simulink model "F550_Attitude_ctrl_SMC"  (R2024a)
settings: Solver=ode4  StartTime=0.0  StopTime=30  FixedStep=0.001  RelTol=1e-3
values from neighbouring files (symbols this model uses):
  r2d = 180/pi    (= 57.2957795131)    [Run_F550_Attitude_Sim.m]    (also in Run_F550_Attitude_Sim_SMC.m)
undefined symbols (not defined in the file or in its folder): Jxx, Jyy, Jzz, SampleTime
libraries: slpidlib x14, simulink x4, simulink_extras x3, matrix_library x1
(part 1 of 2)
settings Model: Creator=ADMIN  LastModifiedBy=UASG
settings DataIOCC: ExternalInput=getinputstruct(op_trim1)  InitialState=getstatestruct(op_trim1)
settings DebuggingCC: UnconnectedInputMsg=warning  UnconnectedOutputMsg=warning  UnconnectedLineMsg=warning  UnderSpecifiedDimensionMsg=warning
settings ModelReferenceCC: EnableRefExpFcnMdlSchedulingChecks=on
settings RTWCC: GPUComputeCapability=3.5  DLArmComputeVersion=19.05

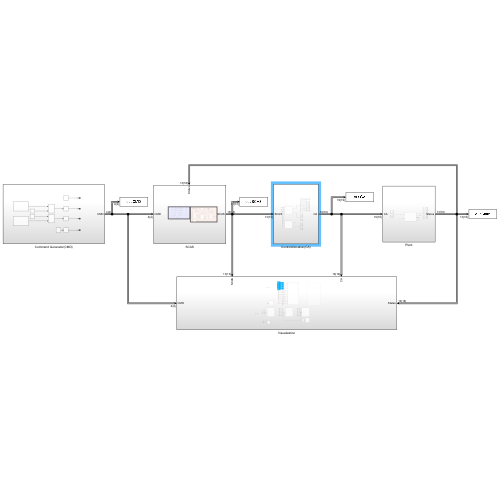
[thumbnail: Simulink's stored preview of the top-level diagram]
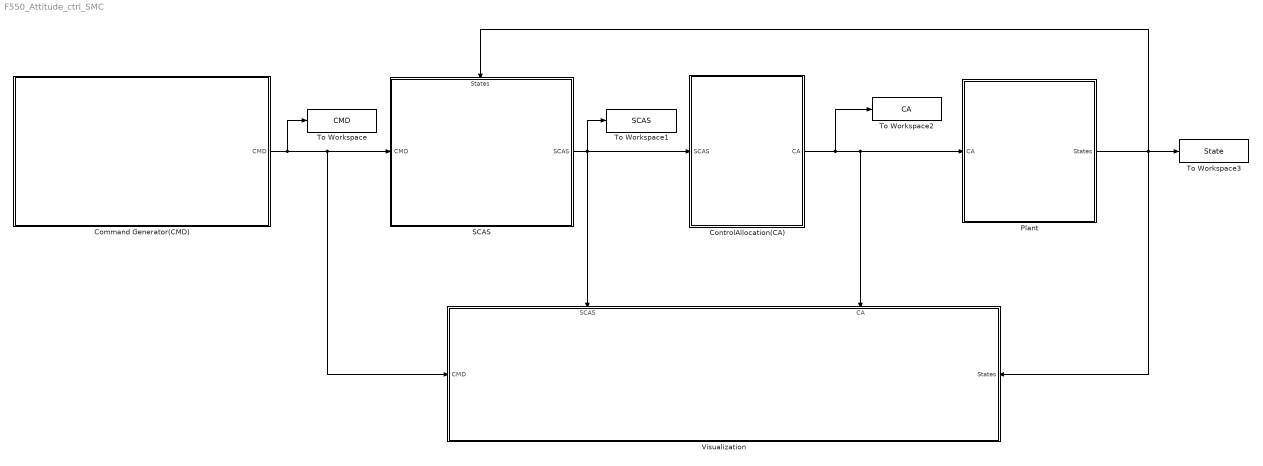
== system F550_Attitude_ctrl_SMC ==
  Command Generator(CMD) : Subsystem
  ControlAllocation(CA) : Subsystem
  Plant : Subsystem
  SCAS : Subsystem
      settings: PortSchema="{\"entries\":[{\"content\":{\"sides\":[{\"content\":{\"connectorIds\":[\"In1\"]},\"type\":\"ConnectorPlacement.EquallySpacedRectSide\",\"uuid\":\"45c0ffbb-c8f4-4882-ae07-b7c3e206befd\"},{\"content\":{\"connectorIds\":[\"Out1\"],\"side\":\"RIGHT\"},\"type\":\"ConnectorPlacement.EquallySpacedRectSide\",\"uuid\":\"fea4074d-042e-40e0-9516-e60d5ceca645\"},{\"content\":{\"connectorIds\":[\"In2\"],\"side\":\"TOP\"},\"type\":\"ConnectorPlacement.EquallySpacedRectSide\",\"uuid\":\"f0d79ab8-0f8c-4372-8ce2-381c487e77f0\"}]},\"type\":\"ConnectorPlacement.EquallySpacedConnector\",\"uuid\":\"9d757277-2882-485b-80f7-2c3f01a5660c\"}],\"packageUris\":[\"http://schema.mathworks.com/mf0/Connector/R2020b\"],\"version\":\"1.0\"}"
  To Workspace : ToWorkspace  VariableName=CMD  SaveFormat=Timeseries  SampleTime=-1
      settings: Save2DSignal=2-D array (concatenate along first dimension)
  To Workspace1 : ToWorkspace  VariableName=SCAS  SaveFormat=Timeseries  SampleTime=-1
      settings: Save2DSignal=2-D array (concatenate along first dimension)
  To Workspace2 : ToWorkspace  VariableName=CA  SaveFormat=Timeseries  SampleTime=-1
      settings: Save2DSignal=2-D array (concatenate along first dimension)
  To Workspace3 : ToWorkspace  VariableName=State  SaveFormat=Timeseries  SampleTime=-1
      settings: Save2DSignal=2-D array (concatenate along first dimension)
  Visualization : Subsystem
      settings: PortSchema="{\"entries\":[{\"content\":{\"sides\":[{\"content\":{\"connectorIds\":[\"In1\"]},\"type\":\"ConnectorPlacement.EquallySpacedRectSide\",\"uuid\":\"45c0ffbb-c8f4-4882-ae07-b7c3e206befd\"},{\"content\":{\"connectorIds\":[\"In4\"],\"side\":\"RIGHT\"},\"type\":\"ConnectorPlacement.EquallySpacedRectSide\",\"uuid\":\"fea4074d-042e-40e0-9516-e60d5ceca645\"},{\"content\":{\"connectorIds\":[\"In2\",\"In3\"],\"side\":\"TOP\"},\"type\":\"ConnectorPlacement.EquallySpacedRectSide\",\"uuid\":\"f0d79ab8-0f8c-4372-8ce2-381c487e77f0\"}]},\"type\":\"ConnectorPlacement.EquallySpacedConnector\",\"uuid\":\"9d757277-2882-485b-80f7-2c3f01a5660c\"}],\"packageUris\":[\"http://schema.mathworks.com/mf0/Connector/R2020b\"],\"version\":\"1.0\"}"
  wires:
  Command Generator(CMD)/1(CMD) -> To Workspace/1, Visualization/1(CMD), SCAS/1(CMD)
  Plant/1(States) -> SCAS/2(States), To Workspace3/1, Visualization/4(States)
  SCAS/1(SCAS) -> To Workspace1/1, ControlAllocation(CA)/1(SCAS), Visualization/2(SCAS)
  ControlAllocation(CA)/1(CA) -> To Workspace2/1, Visualization/3(CA), Plant/1(CA)

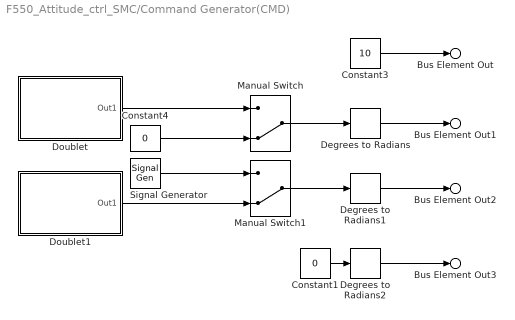
== system F550_Attitude_ctrl_SMC/Command Generator(CMD) ==
  Constant1 : Constant  Value=0
  Constant3 : Constant  Value=10
  Constant4 : Constant  Value=0
  Degrees to Radians : simulink_extras/Transformations/Degrees to Radians
  Degrees to Radians1 : simulink_extras/Transformations/Degrees to Radians
  Degrees to Radians2 : simulink_extras/Transformations/Degrees to Radians
  Doublet : Subsystem
  Doublet1 : Subsystem
  Manual Switch : ManualSwitch  CurrentSetting=0
  Manual Switch1 : ManualSwitch  CurrentSetting=0
  Signal Generator : SignalGenerator  Amplitude=10  Frequency=0.5
  Bus Element Out : Outport  PortName=CMD  Element=des_altitude
  Bus Element Out1 : Outport  PortName=CMD  Element=des_pitch
  Bus Element Out2 : Outport  PortName=CMD  Element=des_roll
  Bus Element Out3 : Outport  PortName=CMD  Element=des_yawrate
  wires:
  Constant1/1 -> Degrees to Radians2/1
  Degrees to Radians2/1 -> Bus Element Out3/1
  Constant3/1 -> Bus Element Out/1
  Degrees to Radians1/1 -> Bus Element Out2/1
  Degrees to Radians/1 -> Bus Element Out1/1
  Manual Switch/1 -> Degrees to Radians/1
  Constant4/1 -> Manual Switch/2
  Manual Switch1/1 -> Degrees to Radians1/1
  Signal Generator/1 -> Manual Switch1/1
  Doublet1/1(Out1) -> Manual Switch1/2
  Doublet/1(Out1) -> Manual Switch/1

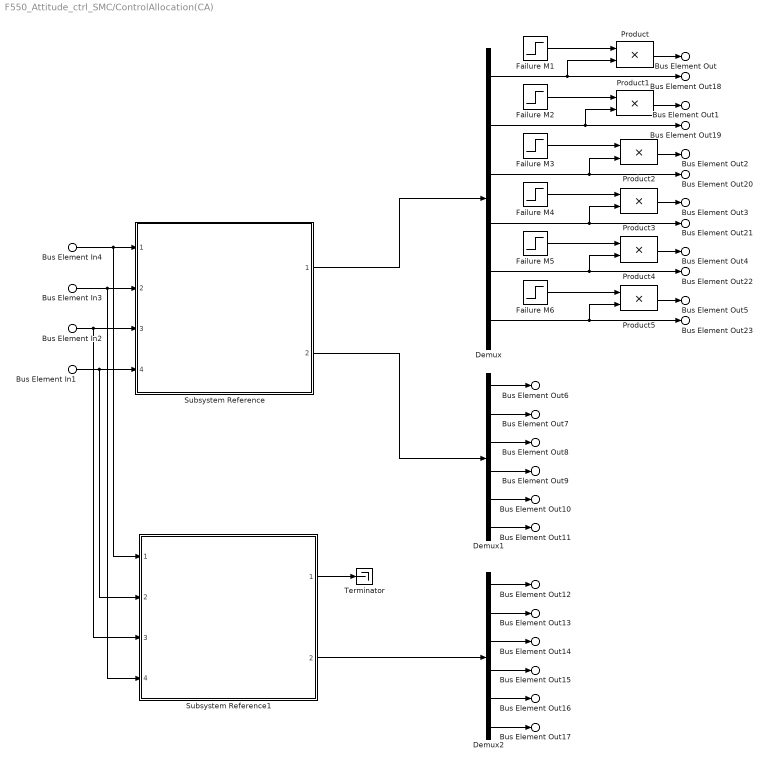
== system F550_Attitude_ctrl_SMC/ControlAllocation(CA) ==
  Bus Element In1 : Inport  PortName=SCAS  Element=tau_roll_smc
  Bus Element In2 : Inport  PortName=SCAS  Element=tau_pitch
  Bus Element In3 : Inport  PortName=SCAS  Element=tau_yaw
  Bus Element In4 : Inport  PortName=SCAS  Element=throttle
  " Failure M3" : Step  Time=23  Before=1  SampleTime=0
  " Failure M4" : Step  Time=23  Before=1  SampleTime=0
  " Failure M5" : Step  Time=23  Before=1  SampleTime=0
  " Failure M6 " : Step  Time=23  Before=1  SampleTime=0
  Demux : Demux  Outputs=6
  Demux1 : Demux  Outputs=6
  Demux2 : Demux  Outputs=6
  Failure M1 : Step  Time=23  Before=1  After=0.5  SampleTime=0
  Failure M2 : Step  Time=23  Before=1  SampleTime=0
  Product{,1..5} (6 alike) : Product
  Subsystem Reference : Subsystem  ReferencedSubsystem=F550_ControlAllocation_sub_ver2023b
  Subsystem Reference1 : Subsystem  ReferencedSubsystem=F550_Adam_CA
  Terminator : Terminator
  Bus Element Out : Outport  PortName=CA  Element=thr_m1
  Bus Element Out1 : Outport  PortName=CA  Element=thr_m2
  Bus Element Out2 : Outport  PortName=CA  Element=thr_m3
  Bus Element Out3 : Outport  PortName=CA  Element=thr_m4
  Bus Element Out4 : Outport  PortName=CA  Element=thr_m5
  Bus Element Out5 : Outport  PortName=CA  Element=thr_m6
  Bus Element Out6 : Outport  PortName=CA  Element=thr_before_saturation_m1
  Bus Element Out7 : Outport  PortName=CA  Element=thr_before_saturation_m2
  Bus Element Out8 : Outport  PortName=CA  Element=thr_before_saturation_m3
  Bus Element Out9 : Outport  PortName=CA  Element=thr_before_saturation_m4
  Bus Element Out10 : Outport  PortName=CA  Element=thr_before_saturation_m5
  Bus Element Out11 : Outport  PortName=CA  Element=thr_before_saturation_m6
  Bus Element Out12 : Outport  PortName=CA  Element=thr_adam_m1
  Bus Element Out13 : Outport  PortName=CA  Element=thr_adam_m2
  Bus Element Out14 : Outport  PortName=CA  Element=thr_adam_m3
  Bus Element Out15 : Outport  PortName=CA  Element=thr_adam_m4
  Bus Element Out16 : Outport  PortName=CA  Element=thr_adam_m5
  Bus Element Out17 : Outport  PortName=CA  Element=thr_adam_m6
  Bus Element Out18 : Outport  PortName=CA  Element=thr_m1_before_fail
  Bus Element Out19 : Outport  PortName=CA  Element=thr_m2_before_fail
  Bus Element Out20 : Outport  PortName=CA  Element=thr_m3_before_fail
  Bus Element Out21 : Outport  PortName=CA  Element=thr_m4_before_fail4
  Bus Element Out22 : Outport  PortName=CA  Element=thr_m5_before_fail
  Bus Element Out23 : Outport  PortName=CA  Element=thr_m6_before_fail
  wires:
  Bus Element In4/1 -> Subsystem Reference1/1, Subsystem Reference/1
  Bus Element In3/1 -> Subsystem Reference1/4, Subsystem Reference/2
  Bus Element In2/1 -> Subsystem Reference1/3, Subsystem Reference/3
  Bus Element In1/1 -> Subsystem Reference1/2, Subsystem Reference/4
  Subsystem Reference/2 -> Demux1/1
  Demux1/1 -> Bus Element Out6/1
  Demux1/2 -> Bus Element Out7/1
  Demux1/3 -> Bus Element Out8/1
  Demux1/4 -> Bus Element Out9/1
  Demux1/5 -> Bus Element Out10/1
  Demux1/6 -> Bus Element Out11/1
  Subsystem Reference1/2 -> Demux2/1
  Subsystem Reference1/1 -> Terminator/1
  Demux2/1 -> Bus Element Out12/1
  Demux2/2 -> Bus Element Out13/1
  Demux2/3 -> Bus Element Out14/1
  Demux2/4 -> Bus Element Out15/1
  Demux2/5 -> Bus Element Out16/1
  Demux2/6 -> Bus Element Out17/1
  Product/1 -> Bus Element Out/1
  Demux/1 -> Bus Element Out18/1, Product/2
  Failure M1/1 -> Product/1
  Subsystem Reference/1 -> Demux/1
  Demux/2 -> Product1/2, Bus Element Out19/1
  Product1/1 -> Bus Element Out1/1
  Failure M2/1 -> Product1/1
  Demux/3 -> Product2/2, Bus Element Out20/1
  Product2/1 -> Bus Element Out2/1
  " Failure M3"/1 -> Product2/1
  Demux/4 -> Bus Element Out21/1, Product3/2
  Product3/1 -> Bus Element Out3/1
  " Failure M4"/1 -> Product3/1
  Demux/5 -> Bus Element Out22/1, Product4/2
  Product4/1 -> Bus Element Out4/1
  " Failure M5"/1 -> Product4/1
  Demux/6 -> Bus Element Out23/1, Product5/2
  Product5/1 -> Bus Element Out5/1
  " Failure M6 "/1 -> Product5/1

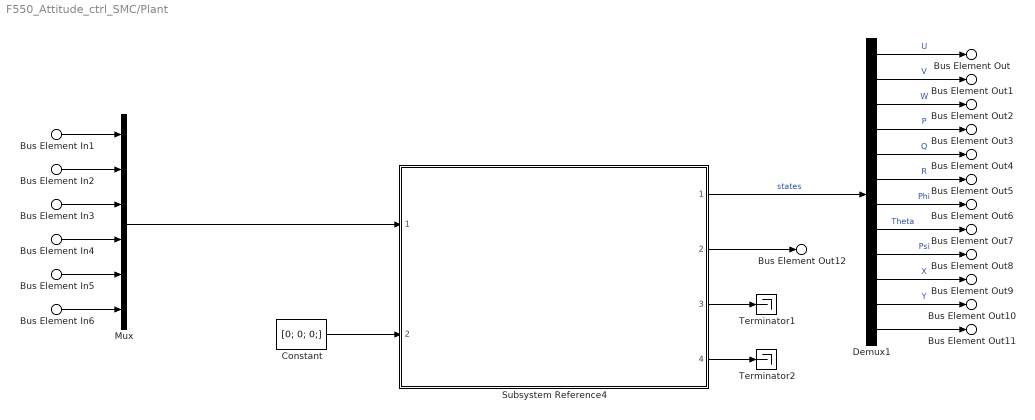
== system F550_Attitude_ctrl_SMC/Plant ==
  Bus Element In1 : Inport  PortName=CA  Element=thr_m1
  Bus Element In2 : Inport  PortName=CA  Element=thr_m2
  Bus Element In3 : Inport  PortName=CA  Element=thr_m3
  Bus Element In4 : Inport  PortName=CA  Element=thr_m4
  Bus Element In5 : Inport  PortName=CA  Element=thr_m5
  Bus Element In6 : Inport  PortName=CA  Element=thr_m6
  Constant : Constant  Value=[0; 0; 0;]
  Demux1 : Demux  Outputs=12
  Mux : Mux  Inputs=6
  Subsystem Reference4 : Subsystem  ReferencedSubsystem=F550_Dynamics_sub_ver2023b
  Terminator1 : Terminator
  Terminator2 : Terminator
  Bus Element Out : Outport  PortName=States  Element=u
  Bus Element Out1 : Outport  PortName=States  Element=v
  Bus Element Out2 : Outport  PortName=States  Element=w
  Bus Element Out3 : Outport  PortName=States  Element=p
  Bus Element Out4 : Outport  PortName=States  Element=q
  Bus Element Out5 : Outport  PortName=States  Element=r
  Bus Element Out6 : Outport  PortName=States  Element=phi
  Bus Element Out7 : Outport  PortName=States  Element=theta
  Bus Element Out8 : Outport  PortName=States  Element=psi
  Bus Element Out9 : Outport  PortName=States  Element=x
  Bus Element Out10 : Outport  PortName=States  Element=y
  Bus Element Out11 : Outport  PortName=States  Element=z
  Bus Element Out12 : Outport  PortName=States  Element=rpm
  wires:
  Subsystem Reference4/1 -> Demux1/1  "states"
  Demux1/1 -> Bus Element Out/1  "U"
  Demux1/2 -> Bus Element Out1/1  "V"
  Demux1/3 -> Bus Element Out2/1  "W"
  Demux1/4 -> Bus Element Out3/1  "P"
  Demux1/5 -> Bus Element Out4/1  "Q"
  Demux1/6 -> Bus Element Out5/1  "R"
  Demux1/7 -> Bus Element Out6/1  "Phi"
  Demux1/8 -> Bus Element Out7/1  "Theta"
  Demux1/9 -> Bus Element Out8/1  "Psi"
  Demux1/10 -> Bus Element Out9/1  "X"
  Demux1/11 -> Bus Element Out10/1  "Y"
  Demux1/12 -> Bus Element Out11/1
  Subsystem Reference4/2 -> Bus Element Out12/1
  Subsystem Reference4/3 -> Terminator1/1
  Subsystem Reference4/4 -> Terminator2/1
  Bus Element In1/1 -> Mux/1
  Bus Element In2/1 -> Mux/2
  Bus Element In3/1 -> Mux/3
  Bus Element In4/1 -> Mux/4
  Bus Element In5/1 -> Mux/5
  Bus Element In6/1 -> Mux/6
  Mux/1 -> Subsystem Reference4/1
  Constant/1 -> Subsystem Reference4/2

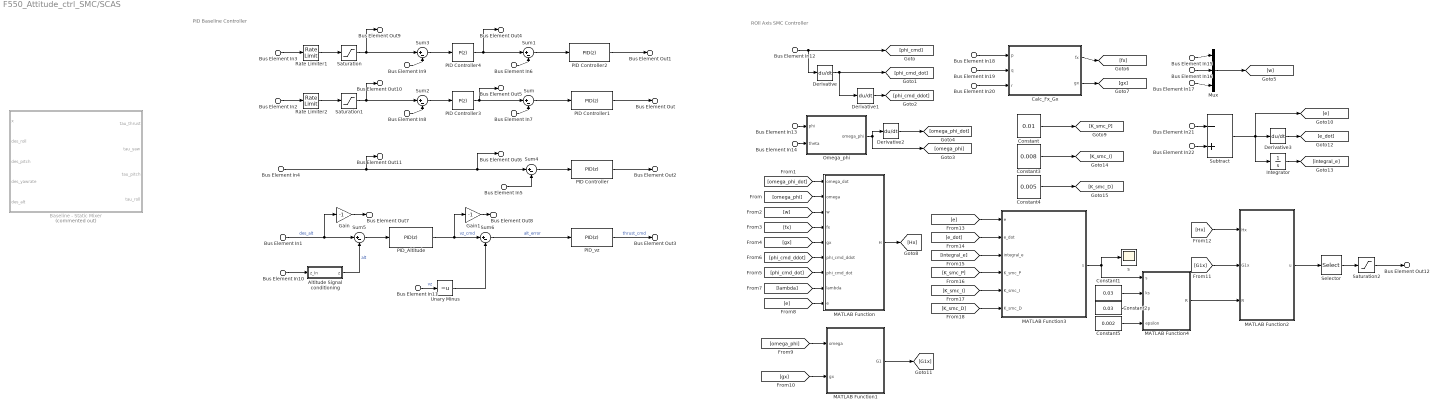
== system F550_Attitude_ctrl_SMC/SCAS ==
  note: ROll Axis SMC Controller
  note: PID Baseline Controller
  Bus Element In1 : Inport  PortName=CMD  Element=des_altitude
  Bus Element In2 : Inport  PortName=CMD  Element=des_pitch
  Bus Element In3 : Inport  PortName=CMD  Element=des_roll
  Bus Element In12 : Inport  PortName=CMD  Element=des_roll
  Bus Element In21 : Inport  PortName=CMD  Element=des_roll
  Bus Element In4 : Inport  PortName=CMD  Element=des_yawrate
  Bus Element In5 : Inport  Port=2  PortName=States  Element=r
  Bus Element In17 : Inport  Port=2  PortName=States  Element=r
  Bus Element In20 : Inport  Port=2  PortName=States  Element=r
  Bus Element In6 : Inport  Port=2  PortName=States  Element=p
  Bus Element In15 : Inport  Port=2  PortName=States  Element=p
  Bus Element In18 : Inport  Port=2  PortName=States  Element=p
  Bus Element In7 : Inport  Port=2  PortName=States  Element=q
  Bus Element In16 : Inport  Port=2  PortName=States  Element=q
  Bus Element In19 : Inport  Port=2  PortName=States  Element=q
  Bus Element In8 : Inport  Port=2  PortName=States  Element=theta
  Bus Element In14 : Inport  Port=2  PortName=States  Element=theta
  Bus Element In9 : Inport  Port=2  PortName=States  Element=phi
  Bus Element In13 : Inport  Port=2  PortName=States  Element=phi
  Bus Element In22 : Inport  Port=2  PortName=States  Element=phi
  Bus Element In10 : Inport  Port=2  PortName=States  Element=z
  Bus Element In11 : Inport  Port=2  PortName=States  Element=w
  Altitude Signal conditioning : Subsystem
  Baseline - Static Mixer : Subsystem  Commented=on
  Calc_Fx_Gx : Subsystem
  Constant : Constant  Value=0.01
  Constant1 : Constant  Value=0.03
  Constant2 : Constant  Value=0.03
  Constant3 : Constant  Value=0.008
  Constant4 : Constant  Value=0.005
  Constant5 : Constant  Value=0.002
  Derivative{,1..3} (4 alike) : Derivative
  Gain : Gain  Gain=-1
  Gain1 : Gain  Gain=-1
  Integrator : Integrator
  MATLAB Function : MATLAB Function  TreatAsAtomicUnit=on
  MATLAB Function1 : MATLAB Function  TreatAsAtomicUnit=on
  MATLAB Function2 : MATLAB Function  TreatAsAtomicUnit=on
  MATLAB Function3 : MATLAB Function  TreatAsAtomicUnit=on
  MATLAB Function4 : MATLAB Function  TreatAsAtomicUnit=on
  Mux : Mux  Inputs=3
  Omega_phi : MATLAB Function  TreatAsAtomicUnit=on
  PID Controller : slpidlib/PID Controller  Controller=PID  Form=Parallel  TimeDomain=Discrete-time  UseExternalTs=off  SampleTime=-1  IntegratorMethod=Forward Euler  FilterMethod=Forward Euler  ControllerParametersSource=internal  P=0.2  I=0.1  UseKiTs=off  D=0  UseExternalDerivativeSource=off  N=100  UseFilter=on  TunerSelectOption=Transfer Function Based (PID Tuner App)  InitialConditionSource=internal  InitialConditionForIntegrator=0  InitialConditionForFilter=0  DifferentiatorICPrevScaledInput=0  ExternalReset=none  TrackingMode=off  Kt=1  LimitOutput=off  SatLimitsSource=internal  UpperSaturationLimit=0.1  LowerSaturationLimit=-0.1  LinearizeAsGain=on  AntiWindupMode=clamping  Kb=1  LimitIntegrator=off  UpperIntegratorSaturationLimit=inf  LowerIntegratorSaturationLimit=-inf  POutMin=[]  POutMax=[]  IOutMin=[]  IOutMax=[]  DOutMin=[]  DOutMax=[]  NOutMin=[]  NOutMax=[]  SumOutMin=[]  SumOutMax=[]  SaturationOutMin=[]  SaturationOutMax=[]  PParamMin=[]  PParamMax=[]  IParamMin=[]  IParamMax=[]  DParamMin=[]  DParamMax=[]  NParamMin=[]  NParamMax=[]  KbParamMin=[]  KbParamMax=[]  KtParamMin=[]  KtParamMax=[]  KbOutMin=[]  KbOutMax=[]  KtOutMin=[]  KtOutMax=[]  IntegratorOutMin=[]  IntegratorOutMax=[]  FilterOutMin=[]  FilterOutMax=[]  SumI1OutMin=[]  SumI1OutMax=[]  SumI2OutMin=[]  SumI2OutMax=[]  SumI3OutMin=[]  SumI3OutMax=[]  SumI4OutMin=[]  SumI4OutMax=[]  SumDOutMin=[]  SumDOutMax=[]  DifferentiatorOutMin=[]  DifferentiatorOutMax=[]  FilterDiffOutCoefMin=[]  FilterDiffOutCoefMax=[]  ReciprocalOutMin=[]  ReciprocalOutMax=[]  SumDenOutMin=[]  SumDenOutMax=[]  SumNumOutMin=[]  SumNumOutMax=[]  DivideOutMin=[]  DivideOutMax=[]  UdiffTsProdOutMin=[]  UdiffTsProdOutMax=[]  NTsProdOutMin=[]  NTsProdOutMax=[]  UintegralTsProdOutMin=[]  UintegralTsProdOutMax=[]  UngainTsProdOutMin=[]  UngainTsProdOutMax=[]  ClampingZeroOutDataTypeStr=Inherit: Inherit via back propagation  ClampingZeroOutMin=[]  ClampingZeroOutMax=[]  FilterDenConstantOutDataTypeStr=Inherit: Inherit via back propagation  FilterDenConstantOutMin=[]  FilterDenConstantOutMax=[]  PCopyOutDataTypeStr=Inherit: Inherit via back propagation  PCopyOutMin=[]  PCopyOutMax=[]  NCopyOutDataTypeStr=Inherit: Inherit via back propagation  NCopyOutMin=[]  NCopyOutMax=[]  IntegratorContinuousStateAttributes=''  IntegratorStateMustResolveToSignalObject=off  IntegratorRTWStateStorageClass=Auto  FilterContinuousStateAttributes=''  FilterStateMustResolveToSignalObject=off  FilterRTWStateStorageClass=Auto  ParallelPVariant=InternalParameters  IdealPVariant=Disabled  IVariant=InternalParameters  DVariant=InternalParameters  IntegratorVariant=Discrete  SatVariant=Disabled  AWVariant=Passthrough  PCopyVariant=Disabled  TRVariant=Disabled  FdbkBlocksVariant=Forward  IdealPFdbkVariant=Disabled  SatFdbkVariant=Disabled  DerivativeFilterVariant=ForwardEulerFilter  NVariant=InternalParameters  NCopyVariant=Disabled  FilterICVariant=InternalICsFilter  IntegratorICVariant=InternalICs  ExternalResetVariant=Disabled  TRSumVariant=Passthrough  SumFdbkVariant=Disabled  SumVariant=Sum_PID  TsampFilterVariant=InternalTs  TsampNgainVariant=Passthrough  TsampIntegralVariant=Disabled_SignalSpec  ExternalSaturationOutDataTypeStr=Inherit: Same as second input  DerivativeSourceVariant=ErrorSignal
  PID Controller1 : slpidlib/PID Controller  Controller=PID  Form=Parallel  TimeDomain=Discrete-time  UseExternalTs=off  SampleTime=-1  IntegratorMethod=Forward Euler  FilterMethod=Forward Euler  ControllerParametersSource=internal  P=0.17  I=0.2  UseKiTs=off  D=0.006  UseExternalDerivativeSource=off  N=50  UseFilter=on  TunerSelectOption=Transfer Function Based (PID Tuner App)  InitialConditionSource=internal  InitialConditionForIntegrator=0  InitialConditionForFilter=0  DifferentiatorICPrevScaledInput=0  ExternalReset=none  TrackingMode=off  Kt=1  LimitOutput=off  SatLimitsSource=internal  UpperSaturationLimit=0.2  LowerSaturationLimit=-0.2  LinearizeAsGain=on  AntiWindupMode=clamping  Kb=1  LimitIntegrator=off  UpperIntegratorSaturationLimit=inf  LowerIntegratorSaturationLimit=-inf  POutMin=[]  POutMax=[]  IOutMin=[]  IOutMax=[]  DOutMin=[]  DOutMax=[]  NOutMin=[]  NOutMax=[]  SumOutMin=[]  SumOutMax=[]  SaturationOutMin=[]  SaturationOutMax=[]  PParamMin=[]  PParamMax=[]  IParamMin=[]  IParamMax=[]  DParamMin=[]  DParamMax=[]  NParamMin=[]  NParamMax=[]  KbParamMin=[]  KbParamMax=[]  KtParamMin=[]  KtParamMax=[]  KbOutMin=[]  KbOutMax=[]  KtOutMin=[]  KtOutMax=[]  IntegratorOutMin=[]  IntegratorOutMax=[]  FilterOutMin=[]  FilterOutMax=[]  SumI1OutMin=[]  SumI1OutMax=[]  SumI2OutMin=[]  SumI2OutMax=[]  SumI3OutMin=[]  SumI3OutMax=[]  SumI4OutMin=[]  SumI4OutMax=[]  SumDOutMin=[]  SumDOutMax=[]  DifferentiatorOutMin=[]  DifferentiatorOutMax=[]  FilterDiffOutCoefMin=[]  FilterDiffOutCoefMax=[]  ReciprocalOutMin=[]  ReciprocalOutMax=[]  SumDenOutMin=[]  SumDenOutMax=[]  SumNumOutMin=[]  SumNumOutMax=[]  DivideOutMin=[]  DivideOutMax=[]  UdiffTsProdOutMin=[]  UdiffTsProdOutMax=[]  NTsProdOutMin=[]  NTsProdOutMax=[]  UintegralTsProdOutMin=[]  UintegralTsProdOutMax=[]  UngainTsProdOutMin=[]  UngainTsProdOutMax=[]  ClampingZeroOutDataTypeStr=Inherit: Inherit via back propagation  ClampingZeroOutMin=[]  ClampingZeroOutMax=[]  FilterDenConstantOutDataTypeStr=Inherit: Inherit via back propagation  FilterDenConstantOutMin=[]  FilterDenConstantOutMax=[]  PCopyOutDataTypeStr=Inherit: Inherit via back propagation  PCopyOutMin=[]  PCopyOutMax=[]  NCopyOutDataTypeStr=Inherit: Inherit via back propagation  NCopyOutMin=[]  NCopyOutMax=[]  IntegratorContinuousStateAttributes=''  IntegratorStateMustResolveToSignalObject=off  IntegratorRTWStateStorageClass=Auto  FilterContinuousStateAttributes=''  FilterStateMustResolveToSignalObject=off  FilterRTWStateStorageClass=Auto  ParallelPVariant=InternalParameters  IdealPVariant=Disabled  IVariant=InternalParameters  DVariant=InternalParameters  IntegratorVariant=Discrete  SatVariant=Disabled  AWVariant=Passthrough  PCopyVariant=Disabled  TRVariant=Disabled  FdbkBlocksVariant=Forward  IdealPFdbkVariant=Disabled  SatFdbkVariant=Disabled  DerivativeFilterVariant=ForwardEulerFilter  NVariant=InternalParameters  NCopyVariant=Disabled  FilterICVariant=InternalICsFilter  IntegratorICVariant=InternalICs  ExternalResetVariant=Disabled  TRSumVariant=Passthrough  SumFdbkVariant=Disabled  SumVariant=Sum_PID  TsampFilterVariant=InternalTs  TsampNgainVariant=Passthrough  TsampIntegralVariant=Disabled_SignalSpec  ExternalSaturationOutDataTypeStr=Inherit: Same as second input  DerivativeSourceVariant=ErrorSignal
  PID Controller2 : slpidlib/PID Controller  Controller=PID  Form=Parallel  TimeDomain=Discrete-time  UseExternalTs=off  SampleTime=-1  IntegratorMethod=Forward Euler  FilterMethod=Forward Euler  ControllerParametersSource=internal  P=0.17  I=0.2  UseKiTs=off  D=0.006  UseExternalDerivativeSource=off  N=50  UseFilter=on  TunerSelectOption=Transfer Function Based (PID Tuner App)  InitialConditionSource=internal  InitialConditionForIntegrator=0  InitialConditionForFilter=0  DifferentiatorICPrevScaledInput=0  ExternalReset=none  TrackingMode=off  Kt=1  LimitOutput=off  SatLimitsSource=internal  UpperSaturationLimit=0.2  LowerSaturationLimit=-0.2  LinearizeAsGain=on  AntiWindupMode=clamping  Kb=1  LimitIntegrator=off  UpperIntegratorSaturationLimit=inf  LowerIntegratorSaturationLimit=-inf  POutMin=[]  POutMax=[]  IOutMin=[]  IOutMax=[]  DOutMin=[]  DOutMax=[]  NOutMin=[]  NOutMax=[]  SumOutMin=[]  SumOutMax=[]  SaturationOutMin=[]  SaturationOutMax=[]  PParamMin=[]  PParamMax=[]  IParamMin=[]  IParamMax=[]  DParamMin=[]  DParamMax=[]  NParamMin=[]  NParamMax=[]  KbParamMin=[]  KbParamMax=[]  KtParamMin=[]  KtParamMax=[]  KbOutMin=[]  KbOutMax=[]  KtOutMin=[]  KtOutMax=[]  IntegratorOutMin=[]  IntegratorOutMax=[]  FilterOutMin=[]  FilterOutMax=[]  SumI1OutMin=[]  SumI1OutMax=[]  SumI2OutMin=[]  SumI2OutMax=[]  SumI3OutMin=[]  SumI3OutMax=[]  SumI4OutMin=[]  SumI4OutMax=[]  SumDOutMin=[]  SumDOutMax=[]  DifferentiatorOutMin=[]  DifferentiatorOutMax=[]  FilterDiffOutCoefMin=[]  FilterDiffOutCoefMax=[]  ReciprocalOutMin=[]  ReciprocalOutMax=[]  SumDenOutMin=[]  SumDenOutMax=[]  SumNumOutMin=[]  SumNumOutMax=[]  DivideOutMin=[]  DivideOutMax=[]  UdiffTsProdOutMin=[]  UdiffTsProdOutMax=[]  NTsProdOutMin=[]  NTsProdOutMax=[]  UintegralTsProdOutMin=[]  UintegralTsProdOutMax=[]  UngainTsProdOutMin=[]  UngainTsProdOutMax=[]  ClampingZeroOutDataTypeStr=Inherit: Inherit via back propagation  ClampingZeroOutMin=[]  ClampingZeroOutMax=[]  FilterDenConstantOutDataTypeStr=Inherit: Inherit via back propagation  FilterDenConstantOutMin=[]  FilterDenConstantOutMax=[]  PCopyOutDataTypeStr=Inherit: Inherit via back propagation  PCopyOutMin=[]  PCopyOutMax=[]  NCopyOutDataTypeStr=Inherit: Inherit via back propagation  NCopyOutMin=[]  NCopyOutMax=[]  IntegratorContinuousStateAttributes=''  IntegratorStateMustResolveToSignalObject=off  IntegratorRTWStateStorageClass=Auto  FilterContinuousStateAttributes=''  FilterStateMustResolveToSignalObject=off  FilterRTWStateStorageClass=Auto  ParallelPVariant=InternalParameters  IdealPVariant=Disabled  IVariant=InternalParameters  DVariant=InternalParameters  IntegratorVariant=Discrete  SatVariant=Disabled  AWVariant=Passthrough  PCopyVariant=Disabled  TRVariant=Disabled  FdbkBlocksVariant=Forward  IdealPFdbkVariant=Disabled  SatFdbkVariant=Disabled  DerivativeFilterVariant=ForwardEulerFilter  NVariant=InternalParameters  NCopyVariant=Disabled  FilterICVariant=InternalICsFilter  IntegratorICVariant=InternalICs  ExternalResetVariant=Disabled  TRSumVariant=Passthrough  SumFdbkVariant=Disabled  SumVariant=Sum_PID  TsampFilterVariant=InternalTs  TsampNgainVariant=Passthrough  TsampIntegralVariant=Disabled_SignalSpec  ExternalSaturationOutDataTypeStr=Inherit: Same as second input  DerivativeSourceVariant=ErrorSignal
  PID Controller3 : slpidlib/PID Controller  Controller=P  Form=Parallel  TimeDomain=Discrete-time  UseExternalTs=off  SampleTime=-1  IntegratorMethod=Forward Euler  FilterMethod=Forward Euler  ControllerParametersSource=internal  P=7.0  I=1  UseKiTs=off  D=0  UseExternalDerivativeSource=off  N=100  UseFilter=on  TunerSelectOption=Transfer Function Based (PID Tuner App)  InitialConditionSource=internal  InitialConditionForIntegrator=0  InitialConditionForFilter=0  DifferentiatorICPrevScaledInput=0  ExternalReset=none  TrackingMode=off  Kt=1  LimitOutput=off  SatLimitsSource=internal  UpperSaturationLimit=inf  LowerSaturationLimit=-inf  LinearizeAsGain=on  AntiWindupMode=none  Kb=1  LimitIntegrator=off  UpperIntegratorSaturationLimit=inf  LowerIntegratorSaturationLimit=-inf  POutMin=[]  POutMax=[]  IOutMin=[]  IOutMax=[]  DOutMin=[]  DOutMax=[]  NOutMin=[]  NOutMax=[]  SumOutMin=[]  SumOutMax=[]  SaturationOutMin=[]  SaturationOutMax=[]  PParamMin=[]  PParamMax=[]  IParamMin=[]  IParamMax=[]  DParamMin=[]  DParamMax=[]  NParamMin=[]  NParamMax=[]  KbParamMin=[]  KbParamMax=[]  KtParamMin=[]  KtParamMax=[]  KbOutMin=[]  KbOutMax=[]  KtOutMin=[]  KtOutMax=[]  IntegratorOutMin=[]  IntegratorOutMax=[]  FilterOutMin=[]  FilterOutMax=[]  SumI1OutMin=[]  SumI1OutMax=[]  SumI2OutMin=[]  SumI2OutMax=[]  SumI3OutMin=[]  SumI3OutMax=[]  SumI4OutMin=[]  SumI4OutMax=[]  SumDOutMin=[]  SumDOutMax=[]  DifferentiatorOutMin=[]  DifferentiatorOutMax=[]  FilterDiffOutCoefMin=[]  FilterDiffOutCoefMax=[]  ReciprocalOutMin=[]  ReciprocalOutMax=[]  SumDenOutMin=[]  SumDenOutMax=[]  SumNumOutMin=[]  SumNumOutMax=[]  DivideOutMin=[]  DivideOutMax=[]  UdiffTsProdOutMin=[]  UdiffTsProdOutMax=[]  NTsProdOutMin=[]  NTsProdOutMax=[]  UintegralTsProdOutMin=[]  UintegralTsProdOutMax=[]  UngainTsProdOutMin=[]  UngainTsProdOutMax=[]  ClampingZeroOutDataTypeStr=Inherit: Inherit via back propagation  ClampingZeroOutMin=[]  ClampingZeroOutMax=[]  FilterDenConstantOutDataTypeStr=Inherit: Inherit via back propagation  FilterDenConstantOutMin=[]  FilterDenConstantOutMax=[]  PCopyOutDataTypeStr=Inherit: Inherit via back propagation  PCopyOutMin=[]  PCopyOutMax=[]  NCopyOutDataTypeStr=Inherit: Inherit via back propagation  NCopyOutMin=[]  NCopyOutMax=[]  IntegratorContinuousStateAttributes=''  IntegratorStateMustResolveToSignalObject=off  IntegratorRTWStateStorageClass=Auto  FilterContinuousStateAttributes=''  FilterStateMustResolveToSignalObject=off  FilterRTWStateStorageClass=Auto  ParallelPVariant=InternalParameters  IdealPVariant=Disabled  IVariant=Disabled  DVariant=Disabled  IntegratorVariant=Disabled  SatVariant=Disabled  AWVariant=Disabled  PCopyVariant=Disabled  TRVariant=Disabled  FdbkBlocksVariant=Forward  IdealPFdbkVariant=Disabled  SatFdbkVariant=Disabled  DerivativeFilterVariant=Disabled  NVariant=Disabled  NCopyVariant=Disabled_SignalSpec  FilterICVariant=Disabled  IntegratorICVariant=Disabled  ExternalResetVariant=Disabled  TRSumVariant=Passthrough  SumFdbkVariant=Disabled  SumVariant=Passthrough_P  TsampFilterVariant=InternalTs  TsampNgainVariant=Passthrough  TsampIntegralVariant=Disabled_SignalSpec  ExternalSaturationOutDataTypeStr=Inherit: Same as second input  DerivativeSourceVariant=Disabled
  PID Controller4 : slpidlib/PID Controller  Controller=P  Form=Parallel  TimeDomain=Discrete-time  UseExternalTs=off  SampleTime=-1  IntegratorMethod=Forward Euler  FilterMethod=Forward Euler  ControllerParametersSource=internal  P=7.0  I=1  UseKiTs=off  D=0  UseExternalDerivativeSource=off  N=100  UseFilter=on  TunerSelectOption=Transfer Function Based (PID Tuner App)  InitialConditionSource=internal  InitialConditionForIntegrator=0  InitialConditionForFilter=0  DifferentiatorICPrevScaledInput=0  ExternalReset=none  TrackingMode=off  Kt=1  LimitOutput=off  SatLimitsSource=internal  UpperSaturationLimit=inf  LowerSaturationLimit=-inf  LinearizeAsGain=on  AntiWindupMode=none  Kb=1  LimitIntegrator=off  UpperIntegratorSaturationLimit=inf  LowerIntegratorSaturationLimit=-inf  POutMin=[]  POutMax=[]  IOutMin=[]  IOutMax=[]  DOutMin=[]  DOutMax=[]  NOutMin=[]  NOutMax=[]  SumOutMin=[]  SumOutMax=[]  SaturationOutMin=[]  SaturationOutMax=[]  PParamMin=[]  PParamMax=[]  IParamMin=[]  IParamMax=[]  DParamMin=[]  DParamMax=[]  NParamMin=[]  NParamMax=[]  KbParamMin=[]  KbParamMax=[]  KtParamMin=[]  KtParamMax=[]  KbOutMin=[]  KbOutMax=[]  KtOutMin=[]  KtOutMax=[]  IntegratorOutMin=[]  IntegratorOutMax=[]  FilterOutMin=[]  FilterOutMax=[]  SumI1OutMin=[]  SumI1OutMax=[]  SumI2OutMin=[]  SumI2OutMax=[]  SumI3OutMin=[]  SumI3OutMax=[]  SumI4OutMin=[]  SumI4OutMax=[]  SumDOutMin=[]  SumDOutMax=[]  DifferentiatorOutMin=[]  DifferentiatorOutMax=[]  FilterDiffOutCoefMin=[]  FilterDiffOutCoefMax=[]  ReciprocalOutMin=[]  ReciprocalOutMax=[]  SumDenOutMin=[]  SumDenOutMax=[]  SumNumOutMin=[]  SumNumOutMax=[]  DivideOutMin=[]  DivideOutMax=[]  UdiffTsProdOutMin=[]  UdiffTsProdOutMax=[]  NTsProdOutMin=[]  NTsProdOutMax=[]  UintegralTsProdOutMin=[]  UintegralTsProdOutMax=[]  UngainTsProdOutMin=[]  UngainTsProdOutMax=[]  ClampingZeroOutDataTypeStr=Inherit: Inherit via back propagation  ClampingZeroOutMin=[]  ClampingZeroOutMax=[]  FilterDenConstantOutDataTypeStr=Inherit: Inherit via back propagation  FilterDenConstantOutMin=[]  FilterDenConstantOutMax=[]  PCopyOutDataTypeStr=Inherit: Inherit via back propagation  PCopyOutMin=[]  PCopyOutMax=[]  NCopyOutDataTypeStr=Inherit: Inherit via back propagation  NCopyOutMin=[]  NCopyOutMax=[]  IntegratorContinuousStateAttributes=''  IntegratorStateMustResolveToSignalObject=off  IntegratorRTWStateStorageClass=Auto  FilterContinuousStateAttributes=''  FilterStateMustResolveToSignalObject=off  FilterRTWStateStorageClass=Auto  ParallelPVariant=InternalParameters  IdealPVariant=Disabled  IVariant=Disabled  DVariant=Disabled  IntegratorVariant=Disabled  SatVariant=Disabled  AWVariant=Disabled  PCopyVariant=Disabled  TRVariant=Disabled  FdbkBlocksVariant=Forward  IdealPFdbkVariant=Disabled  SatFdbkVariant=Disabled  DerivativeFilterVariant=Disabled  NVariant=Disabled  NCopyVariant=Disabled_SignalSpec  FilterICVariant=Disabled  IntegratorICVariant=Disabled  ExternalResetVariant=Disabled  TRSumVariant=Passthrough  SumFdbkVariant=Disabled  SumVariant=Passthrough_P  TsampFilterVariant=InternalTs  TsampNgainVariant=Passthrough  TsampIntegralVariant=Disabled_SignalSpec  ExternalSaturationOutDataTypeStr=Inherit: Same as second input  DerivativeSourceVariant=Disabled
  PID_Altitude : slpidlib/PID Controller  Controller=PID  Form=Parallel  TimeDomain=Discrete-time  UseExternalTs=off  SampleTime=-1  IntegratorMethod=Backward Euler  FilterMethod=Forward Euler  ControllerParametersSource=internal  P=1.5  I=0.01  UseKiTs=off  D=0.01  UseExternalDerivativeSource=off  N=10  UseFilter=on  TunerSelectOption=Transfer Function Based (PID Tuner App)  InitialConditionSource=internal  InitialConditionForIntegrator=0  InitialConditionForFilter=0  DifferentiatorICPrevScaledInput=0  ExternalReset=none  TrackingMode=off  Kt=1  LimitOutput=on  SatLimitsSource=internal  UpperSaturationLimit=2  LowerSaturationLimit=-2  LinearizeAsGain=off  AntiWindupMode=clamping  Kb=1  LimitIntegrator=off  UpperIntegratorSaturationLimit=inf  LowerIntegratorSaturationLimit=-inf  POutMin=[]  POutMax=[]  IOutMin=[]  IOutMax=[]  DOutMin=[]  DOutMax=[]  NOutMin=[]  NOutMax=[]  SumOutMin=[]  SumOutMax=[]  SaturationOutMin=[]  SaturationOutMax=[]  PParamMin=[]  PParamMax=[]  IParamMin=[]  IParamMax=[]  DParamMin=[]  DParamMax=[]  NParamMin=[]  NParamMax=[]  KbParamMin=[]  KbParamMax=[]  KtParamMin=[]  KtParamMax=[]  KbOutMin=[]  KbOutMax=[]  KtOutMin=[]  KtOutMax=[]  IntegratorOutMin=[]  IntegratorOutMax=[]  FilterOutMin=[]  FilterOutMax=[]  SumI1OutMin=[]  SumI1OutMax=[]  SumI2OutMin=[]  SumI2OutMax=[]  SumI3OutMin=[]  SumI3OutMax=[]  SumI4OutMin=[]  SumI4OutMax=[]  SumDOutMin=[]  SumDOutMax=[]  DifferentiatorOutMin=[]  DifferentiatorOutMax=[]  FilterDiffOutCoefMin=[]  FilterDiffOutCoefMax=[]  ReciprocalOutMin=[]  ReciprocalOutMax=[]  SumDenOutMin=[]  SumDenOutMax=[]  SumNumOutMin=[]  SumNumOutMax=[]  DivideOutMin=[]  DivideOutMax=[]  UdiffTsProdOutMin=[]  UdiffTsProdOutMax=[]  NTsProdOutMin=[]  NTsProdOutMax=[]  UintegralTsProdOutMin=[]  UintegralTsProdOutMax=[]  UngainTsProdOutMin=[]  UngainTsProdOutMax=[]  ClampingZeroOutDataTypeStr=Inherit: Inherit via back propagation  ClampingZeroOutMin=[]  ClampingZeroOutMax=[]  FilterDenConstantOutDataTypeStr=Inherit: Inherit via back propagation  FilterDenConstantOutMin=[]  FilterDenConstantOutMax=[]  PCopyOutDataTypeStr=Inherit: Inherit via back propagation  PCopyOutMin=[]  PCopyOutMax=[]  NCopyOutDataTypeStr=Inherit: Inherit via back propagation  NCopyOutMin=[]  NCopyOutMax=[]  IntegratorContinuousStateAttributes=''  IntegratorStateMustResolveToSignalObject=off  IntegratorRTWStateStorageClass=Auto  FilterContinuousStateAttributes=''  FilterStateMustResolveToSignalObject=off  FilterRTWStateStorageClass=Auto  ParallelPVariant=InternalParameters  IdealPVariant=Disabled  IVariant=InternalParameters  DVariant=InternalParameters  IntegratorVariant=Discrete  SatVariant=Enabled  AWVariant=DiscClampingParallel  PCopyVariant=Disabled  TRVariant=Disabled  FdbkBlocksVariant=Feedback  IdealPFdbkVariant=Passthrough  SatFdbkVariant=Passthrough  DerivativeFilterVariant=ForwardEulerFilter  NVariant=InternalParameters  NCopyVariant=Disabled  FilterICVariant=InternalICsFilter  IntegratorICVariant=InternalICs  ExternalResetVariant=Disabled  TRSumVariant=Passthrough  SumFdbkVariant=Enabled  SumVariant=Sum_PID  TsampFilterVariant=InternalTs  TsampNgainVariant=Passthrough  TsampIntegralVariant=Disabled_SignalSpec  ExternalSaturationOutDataTypeStr=Inherit: Same as second input  DerivativeSourceVariant=ErrorSignal
  PID_vz : slpidlib/PID Controller  Controller=PID  Form=Parallel  TimeDomain=Discrete-time  UseExternalTs=off  SampleTime=-1  IntegratorMethod=Backward Euler  FilterMethod=Forward Euler  ControllerParametersSource=internal  P=0.5  I=0.1  UseKiTs=off  D=0.05  UseExternalDerivativeSource=off  N=10  UseFilter=on  TunerSelectOption=Transfer Function Based (PID Tuner App)  InitialConditionSource=internal  InitialConditionForIntegrator=0  InitialConditionForFilter=0  DifferentiatorICPrevScaledInput=0  ExternalReset=none  TrackingMode=off  Kt=1  LimitOutput=on  SatLimitsSource=internal  UpperSaturationLimit=1  LowerSaturationLimit=0  LinearizeAsGain=off  AntiWindupMode=clamping  Kb=1  LimitIntegrator=off  UpperIntegratorSaturationLimit=inf  LowerIntegratorSaturationLimit=-inf  POutMin=[]  POutMax=[]  IOutMin=[]  IOutMax=[]  DOutMin=[]  DOutMax=[]  NOutMin=[]  NOutMax=[]  SumOutMin=[]  SumOutMax=[]  SaturationOutMin=[]  SaturationOutMax=[]  PParamMin=[]  PParamMax=[]  IParamMin=[]  IParamMax=[]  DParamMin=[]  DParamMax=[]  NParamMin=[]  NParamMax=[]  KbParamMin=[]  KbParamMax=[]  KtParamMin=[]  KtParamMax=[]  KbOutMin=[]  KbOutMax=[]  KtOutMin=[]  KtOutMax=[]  IntegratorOutMin=[]  IntegratorOutMax=[]  FilterOutMin=[]  FilterOutMax=[]  SumI1OutMin=[]  SumI1OutMax=[]  SumI2OutMin=[]  SumI2OutMax=[]  SumI3OutMin=[]  SumI3OutMax=[]  SumI4OutMin=[]  SumI4OutMax=[]  SumDOutMin=[]  SumDOutMax=[]  DifferentiatorOutMin=[]  DifferentiatorOutMax=[]  FilterDiffOutCoefMin=[]  FilterDiffOutCoefMax=[]  ReciprocalOutMin=[]  ReciprocalOutMax=[]  SumDenOutMin=[]  SumDenOutMax=[]  SumNumOutMin=[]  SumNumOutMax=[]  DivideOutMin=[]  DivideOutMax=[]  UdiffTsProdOutMin=[]  UdiffTsProdOutMax=[]  NTsProdOutMin=[]  NTsProdOutMax=[]  UintegralTsProdOutMin=[]  UintegralTsProdOutMax=[]  UngainTsProdOutMin=[]  UngainTsProdOutMax=[]  ClampingZeroOutDataTypeStr=Inherit: Inherit via back propagation  ClampingZeroOutMin=[]  ClampingZeroOutMax=[]  FilterDenConstantOutDataTypeStr=Inherit: Inherit via back propagation  FilterDenConstantOutMin=[]  FilterDenConstantOutMax=[]  PCopyOutDataTypeStr=Inherit: Inherit via back propagation  PCopyOutMin=[]  PCopyOutMax=[]  NCopyOutDataTypeStr=Inherit: Inherit via back propagation  NCopyOutMin=[]  NCopyOutMax=[]  IntegratorContinuousStateAttributes=''  IntegratorStateMustResolveToSignalObject=off  IntegratorRTWStateStorageClass=Auto  FilterContinuousStateAttributes=''  FilterStateMustResolveToSignalObject=off  FilterRTWStateStorageClass=Auto  ParallelPVariant=InternalParameters  IdealPVariant=Disabled  IVariant=InternalParameters  DVariant=InternalParameters  IntegratorVariant=Discrete  SatVariant=Enabled  AWVariant=DiscClampingParallel  PCopyVariant=Disabled  TRVariant=Disabled  FdbkBlocksVariant=Feedback  IdealPFdbkVariant=Passthrough  SatFdbkVariant=Passthrough  DerivativeFilterVariant=ForwardEulerFilter  NVariant=InternalParameters  NCopyVariant=Disabled  FilterICVariant=InternalICsFilter  IntegratorICVariant=InternalICs  ExternalResetVariant=Disabled  TRSumVariant=Passthrough  SumFdbkVariant=Enabled  SumVariant=Sum_PID  TsampFilterVariant=InternalTs  TsampNgainVariant=Passthrough  TsampIntegralVariant=Disabled_SignalSpec  ExternalSaturationOutDataTypeStr=Inherit: Same as second input  DerivativeSourceVariant=ErrorSignal
  Rate Limiter1 : RateLimiter  RisingSlewLimit=180*pi/180  FallingSlewLimit=-180*pi/180  SampleTimeMode=inherited
  Rate Limiter2 : RateLimiter  RisingSlewLimit=180*pi/180  FallingSlewLimit=-180*pi/180  SampleTimeMode=inherited
  Saturation : Saturate  UpperLimit=20*pi/180  LowerLimit=-20*pi/180
  Saturation1 : Saturate  UpperLimit=20*pi/180  LowerLimit=-20*pi/180
  Saturation2 : Saturate
  Selector : Selector  InputPortWidth=3  IndexOptions=Index vector (dialog)  Indices=1  OutputSizes=1
  Subtract : Sum  Inputs=-+
  Sum{,1..6} (7 alike) : Sum  Inputs=|+-
  Unary Minus : UnaryMinus
  s : Scope
  Bus Element Out : Outport  PortName=SCAS  Element=tau_pitch
  Bus Element Out1 : Outport  PortName=SCAS  Element=tau_roll
  Bus Element Out2 : Outport  PortName=SCAS  Element=tau_yaw
  Bus Element Out3 : Outport  PortName=SCAS  Element=throttle
  Bus Element Out4 : Outport  PortName=SCAS  Element=p_cmd
  Bus Element Out5 : Outport  PortName=SCAS  Element=q_cmd
  Bus Element Out6 : Outport  PortName=SCAS  Element=r_cmd
  Bus Element Out7 : Outport  PortName=SCAS  Element=z_cmd
  Bus Element Out8 : Outport  PortName=SCAS  Element=w_cmd
  Bus Element Out9 : Outport  PortName=SCAS  Element=phi_cmd
  Bus Element Out10 : Outport  PortName=SCAS  Element=theta_cmd
  Bus Element Out11 : Outport  PortName=SCAS  Element=psi_cmd
  Bus Element Out12 : Outport  PortName=SCAS  Element=tau_roll_smc
  wires:
  Bus Element In2/1 -> Rate Limiter2/1
  Bus Element In4/1 -> Bus Element Out11/1, Bus Element Out6/1, Sum4/1
  Bus Element In3/1 -> Rate Limiter1/1
  PID Controller4/1 -> Bus Element Out4/1, Sum1/1
  Sum3/1 -> PID Controller4/1
  PID Controller1/1 -> Bus Element Out/1
  Saturation1/1 -> Bus Element Out10/1, Sum2/1
  Sum2/1 -> PID Controller3/1
  PID Controller3/1 -> Bus Element Out5/1, Sum/1
  Saturation/1 -> Sum3/1, Bus Element Out9/1
  Rate Limiter2/1 -> Saturation1/1
  Sum/1 -> PID Controller1/1
  Sum1/1 -> PID Controller2/1
  Rate Limiter1/1 -> Saturation/1
  PID Controller/1 -> Bus Element Out2/1
  Sum4/1 -> PID Controller/1
  Gain/1 -> Bus Element Out7/1
  Bus Element In11/1 -> Unary Minus/1  "vz"
  Gain1/1 -> Bus Element Out8/1
  Unary Minus/1 -> Sum6/2
  Altitude Signal conditioning/1(z) -> Sum5/2  "alt"
  Sum6/1 -> PID_vz/1  "alt_error"
  Bus Element In1/1 -> Gain/1, Sum5/1  "des_alt"
  Bus Element In10/1 -> Altitude Signal conditioning/1(z_In)
  Sum5/1 -> PID_Altitude/1
  PID_Altitude/1 -> Gain1/1, Sum6/1  "vz_cmd"
  PID_vz/1 -> Bus Element Out3/1  "thrust_cmd"
  Bus Element In5/1 -> Sum4/2
  Bus Element In6/1 -> Sum1/2
  Bus Element In7/1 -> Sum/2
  Bus Element In8/1 -> Sum2/2
  Bus Element In9/1 -> Sum3/2
  Bus Element In12/1 -> [phi_cmd], Derivative/1
  Derivative/1 -> [phi_cmd_dot], Derivative1/1
  Derivative1/1 -> [phi_cmd_ddot]
  Bus Element In13/1 -> Omega_phi/1(phi)
  Bus Element In14/1 -> Omega_phi/2(theta)
  Omega_phi/1(omega_phi) -> Derivative2/1, [omega_phi]
  Derivative2/1 -> [omega_phi_dot]
  Bus Element In15/1 -> Mux/1
  Bus Element In16/1 -> Mux/2
  Bus Element In17/1 -> Mux/3
  Mux/1 -> [w]
  Bus Element In18/1 -> Calc_Fx_Gx/1(p)
  Bus Element In19/1 -> Calc_Fx_Gx/2(q)
  Bus Element In20/1 -> Calc_Fx_Gx/3(r)
  Calc_Fx_Gx/1(fx) -> [fx]
  Calc_Fx_Gx/2(gx) -> [gx]
  MATLAB Function/1(H) -> [Hx]
  [omega_phi_dot] -> MATLAB Function/1(omega_dot)
  [omega_phi] -> MATLAB Function/2(omega)
  [w] -> MATLAB Function/3(w)
  [fx] -> MATLAB Function/4(fx)
  [gx] -> MATLAB Function/5(gx)
  [phi_cmd_ddot] -> MATLAB Function/6(phi_cmd_ddot)
  [phi_cmd_dot] -> MATLAB Function/7(phi_cmd_dot)
  Constant/1 -> [K_smc_P]
  [lambda] -> MATLAB Function/8(lambda)
  Bus Element In21/1 -> Subtract/1
  Bus Element In22/1 -> Subtract/2
  Subtract/1 -> Integrator/1, Derivative3/1, [e]
  [e] -> MATLAB Function/9(e)
  MATLAB Function1/1(G1) -> [G1x]
  [omega_phi] -> MATLAB Function1/1(omega)
  [gx] -> MATLAB Function1/2(gx)
  [G1x] -> MATLAB Function2/2(G1x)
  [Hx] -> MATLAB Function2/1(Hx)
  Derivative3/1 -> [e_dot]
  MATLAB Function3/1(s) -> MATLAB Function4/1(s), s/1
  MATLAB Function4/1(R) -> MATLAB Function2/3(R)
  [e] -> MATLAB Function3/1(e)
  [e_dot] -> MATLAB Function3/2(e_dot)
  Integrator/1 -> [integral_e]
  [integral_e] -> MATLAB Function3/3(integral_e)
  [K_smc_P] -> MATLAB Function3/4(K_smc_P)
  Constant1/1 -> MATLAB Function4/2(ks)
  Constant2/1 -> MATLAB Function4/3(kp)
  MATLAB Function2/1(u) -> Selector/1
  Selector/1 -> Saturation2/1
  Constant3/1 -> [K_smc_I]
  Constant4/1 -> [K_smc_D]
  [K_smc_I] -> MATLAB Function3/5(K_smc_I)
  [K_smc_D] -> MATLAB Function3/6(K_smc_D)
  Saturation2/1 -> Bus Element Out12/1
  Constant5/1 -> MATLAB Function4/4(epsilon)
  PID Controller2/1 -> Bus Element Out1/1

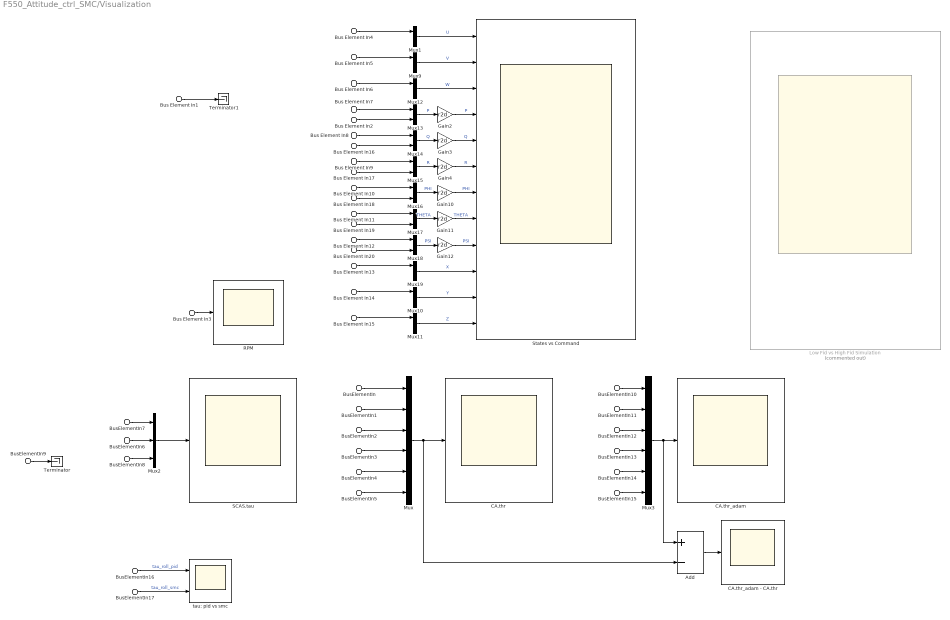
== system F550_Attitude_ctrl_SMC/Visualization ==
  Bus Element In1 : Inport  PortName=CMD  Element=des_yawrate
  Bus Element In2 : Inport  Port=2  PortName=SCAS  Element=p_cmd
  Bus Element In16 : Inport  Port=2  PortName=SCAS  Element=q_cmd
  Bus Element In17 : Inport  Port=2  PortName=SCAS  Element=r_cmd
  Bus Element In18 : Inport  Port=2  PortName=SCAS  Element=phi_cmd
  Bus Element In19 : Inport  Port=2  PortName=SCAS  Element=theta_cmd
  Bus Element In20 : Inport  Port=2  PortName=SCAS  Element=psi_cmd
  BusElementIn6 : Inport  Port=2  PortName=SCAS  Element=tau_pitch
  BusElementIn7 : Inport  Port=2  PortName=SCAS  Element=tau_roll
  BusElementIn16 : Inport  Port=2  PortName=SCAS  Element=tau_roll
  BusElementIn8 : Inport  Port=2  PortName=SCAS  Element=tau_yaw
  BusElementIn9 : Inport  Port=2  PortName=SCAS  Element=throttle
  BusElementIn17 : Inport  Port=2  PortName=SCAS  Element=tau_roll_smc
  BusElementIn : Inport  Port=3  PortName=CA  Element=thr_m1_before_fail
  BusElementIn1 : Inport  Port=3  PortName=CA  Element=thr_m2
  BusElementIn2 : Inport  Port=3  PortName=CA  Element=thr_m3
  BusElementIn3 : Inport  Port=3  PortName=CA  Element=thr_m4
  BusElementIn4 : Inport  Port=3  PortName=CA  Element=thr_m5
  BusElementIn5 : Inport  Port=3  PortName=CA  Element=thr_m6
  BusElementIn10 : Inport  Port=3  PortName=CA  Element=thr_adam_m1
  BusElementIn11 : Inport  Port=3  PortName=CA  Element=thr_adam_m2
  BusElementIn12 : Inport  Port=3  PortName=CA  Element=thr_adam_m3
  BusElementIn13 : Inport  Port=3  PortName=CA  Element=thr_adam_m4
  BusElementIn14 : Inport  Port=3  PortName=CA  Element=thr_adam_m5
  BusElementIn15 : Inport  Port=3  PortName=CA  Element=thr_adam_m6
  Bus Element In4 : Inport  Port=4  PortName=States  Element=u
  Bus Element In5 : Inport  Port=4  PortName=States  Element=v
  Bus Element In6 : Inport  Port=4  PortName=States  Element=w
  Bus Element In7 : Inport  Port=4  PortName=States  Element=p
  Bus Element In8 : Inport  Port=4  PortName=States  Element=q
  Bus Element In9 : Inport  Port=4  PortName=States  Element=r
  Bus Element In10 : Inport  Port=4  PortName=States  Element=phi
  Bus Element In11 : Inport  Port=4  PortName=States  Element=theta
  Bus Element In12 : Inport  Port=4  PortName=States  Element=psi
  Bus Element In13 : Inport  Port=4  PortName=States  Element=x
  Bus Element In14 : Inport  Port=4  PortName=States  Element=y
  Bus Element In15 : Inport  Port=4  PortName=States  Element=z
  Bus Element In3 : Inport  Port=4  PortName=States  Element=rpm
  Add : Sum  Inputs=+-
  CA.thr : Scope
  CA.thr_adam : Scope
  CA.thr_adam - CA.thr : Scope
  Gain{2..4,10..12} (6 alike) : Gain  Gain=r2d
  Low Fid vs High Fid Simulation : Scope  Commented=on  NumInputPorts=12
  Mux : Mux  Inputs=6
  Mux{1,9..19} (12 alike) : Mux  Inputs=2
  Mux2 : Mux  Inputs=3
  Mux3 : Mux  Inputs=6
  RPM : Scope
  SCAS.tau : Scope
  States vs Command : Scope  NumInputPorts=12
  Terminator : Terminator
  Terminator1 : Terminator
  tau: pid vs smc : Scope  NumInputPorts=2
  wires:
  Bus Element In2/1 -> Mux13/2
  ? -> Mux12/2
  Bus Element In8/1 -> Mux14/1
  Mux19/1 -> States vs Command/10  "X"
  Mux15/1 -> Gain4/1  "R"
  Mux1/1 -> States vs Command/1  "U"
  Bus Element In18/1 -> Mux16/2
  Bus Element In19/1 -> Mux17/2
  ? -> Mux1/2
  Bus Element In14/1 -> Mux10/1
  Mux13/1 -> Gain2/1  "P"
  Bus Element In15/1 -> Mux11/1
  Mux10/1 -> States vs Command/11  "Y"
  Bus Element In16/1 -> Mux14/2
  ? -> Mux9/2
  ? -> Mux19/2
  Bus Element In4/1 -> Mux1/1
  Bus Element In7/1 -> Mux13/1
  ? -> Mux10/2
  Bus Element In13/1 -> Mux19/1
  Bus Element In6/1 -> Mux12/1
  Mux16/1 -> Gain10/1  "PHI"
  Mux9/1 -> States vs Command/2  "V"
  Mux14/1 -> Gain3/1  "Q"
  ? -> Mux11/2
  Mux17/1 -> Gain11/1  "THETA"
  Bus Element In20/1 -> Mux18/2
  Bus Element In17/1 -> Mux15/2
  Bus Element In11/1 -> Mux17/1
  Bus Element In10/1 -> Mux16/1
  Bus Element In12/1 -> Mux18/1
  Mux12/1 -> States vs Command/3  "W"
  Mux11/1 -> States vs Command/12  "Z"
  Bus Element In9/1 -> Mux15/1
  Mux18/1 -> Gain12/1  "PSI"
  Gain2/1 -> States vs Command/4  "P"
  Gain3/1 -> States vs Command/5  "Q"
  Gain4/1 -> States vs Command/6  "R"
  Gain10/1 -> States vs Command/7  "PHI"
  Gain11/1 -> States vs Command/8  "THETA"
  Gain12/1 -> States vs Command/9  "PSI"
  Bus Element In5/1 -> Mux9/1
  Bus Element In1/1 -> Terminator1/1
  BusElementIn/1 -> Mux/1
  BusElementIn1/1 -> Mux/2
  BusElementIn2/1 -> Mux/3
  BusElementIn3/1 -> Mux/4
  BusElementIn4/1 -> Mux/5
  BusElementIn5/1 -> Mux/6
  Mux/1 -> Add/2, CA.thr/1
  BusElementIn8/1 -> Mux2/3
  BusElementIn6/1 -> Mux2/2
  BusElementIn7/1 -> Mux2/1
  Mux2/1 -> SCAS.tau/1
  BusElementIn9/1 -> Terminator/1
  Mux3/1 -> Add/1, CA.thr_adam/1
  BusElementIn10/1 -> Mux3/1
  BusElementIn11/1 -> Mux3/2
  BusElementIn15/1 -> Mux3/6
  BusElementIn14/1 -> Mux3/5
  BusElementIn13/1 -> Mux3/4
  BusElementIn12/1 -> Mux3/3
  Add/1 -> CA.thr_adam - CA.thr/1
  BusElementIn16/1 -> tau: pid vs smc/1  "tau_roll_pid"
  BusElementIn17/1 -> tau: pid vs smc/2  "tau_roll_smc"
  Bus Element In3/1 -> RPM/1

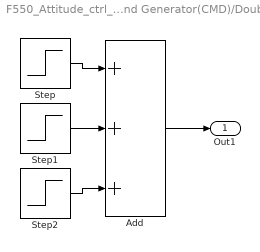
== system F550_Attitude_ctrl_SMC/Command Generator(CMD)/Doublet ==
  Add : Sum  Inputs=+++
  Step : Step  Time=10  After=8  SampleTime=0
  Step1 : Step  Time=15  After=-16  SampleTime=0
  Step2 : Step  Time=20  After=8  SampleTime=0
  Out1 : Outport
  wires:
  Step/1 -> Add/1
  Step1/1 -> Add/2
  Add/1 -> Out1/1
  Step2/1 -> Add/3

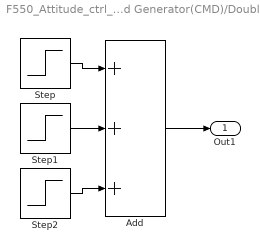
== system F550_Attitude_ctrl_SMC/Command Generator(CMD)/Doublet1 ==
  Add : Sum  Inputs=+++
  Step : Step  Time=10  After=8  SampleTime=0
  Step1 : Step  Time=15  After=-16  SampleTime=0
  Step2 : Step  Time=20  After=8  SampleTime=0
  Out1 : Outport
  wires:
  Step/1 -> Add/1
  Step1/1 -> Add/2
  Add/1 -> Out1/1
  Step2/1 -> Add/3

== system F550_Attitude_ctrl_SMC/SCAS/Altitude Signal conditioning ==
  z_In : Inport
  Constant : Constant  Value=0
  Gain1 : Gain  Gain=-1
  Saturation Dynamic : simulink/Discontinuities/Saturation Dynamic  OutMin=[]  OutMax=[]  OutDataTypeStr=Inherit: Same as second input  OutDataType=fixdt(1, 16)  OutScaling=2^-10  DoSatur=off
  z : Outport
  wires:
  z_In/1 -> Gain1/1
  Gain1/1 -> Saturation Dynamic/1, Saturation Dynamic/2
  Constant/1 -> Saturation Dynamic/3
  Saturation Dynamic/1 -> z/1  "alt"

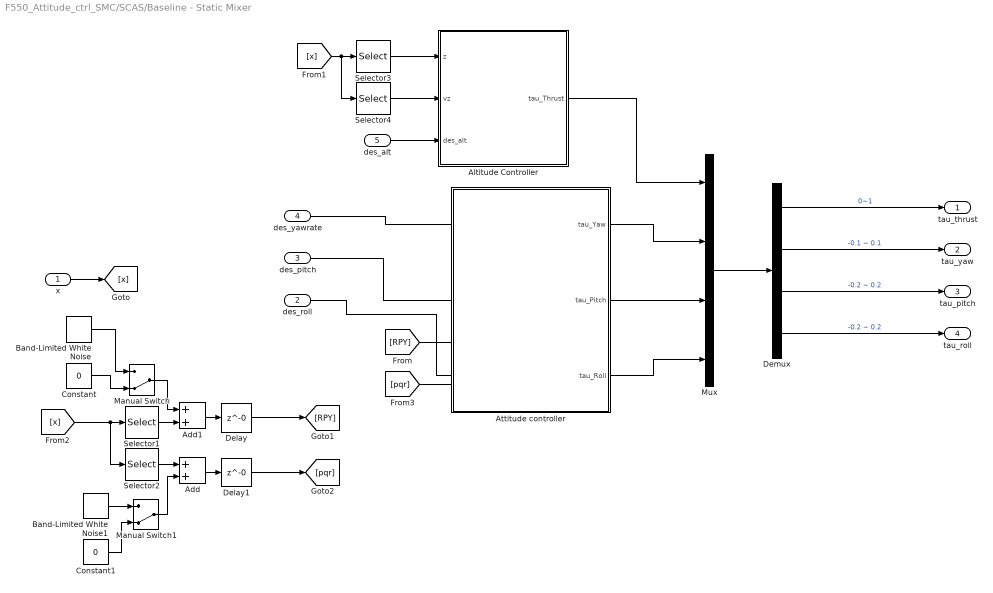
== system F550_Attitude_ctrl_SMC/SCAS/Baseline - Static Mixer ==
  x : Inport
  des_roll : Inport  Port=2
  des_pitch : Inport  Port=3
  des_yawrate : Inport  Port=4
  des_alt : Inport  Port=5
  Add : Sum
  Add1 : Sum
  Altitude Controller : Subsystem
  Attitude controller : Subsystem
  Band-Limited White Noise : simulink/Sources/Band-Limited White Noise  Cov=[1e-5]  Ts=SampleTime  seed=[23341]
  Band-Limited White Noise1 : simulink/Sources/Band-Limited White Noise  Cov=[1e-6]  Ts=SampleTime  seed=[23341]
  Constant : Constant  Value=0
  Constant1 : Constant  Value=0
  Delay : Delay  DelayLength=0
  Delay1 : Delay  DelayLength=0
  Demux : Demux
  Manual Switch : ManualSwitch  CurrentSetting=0
  Manual Switch1 : ManualSwitch  CurrentSetting=0
  Mux : Mux
  Selector1 : Selector  InputPortWidth=12  IndexOptions=Index vector (dialog)  Indices=[7 8 9]  OutputSizes=1
  Selector2 : Selector  InputPortWidth=12  IndexOptions=Index vector (dialog)  Indices=[4 5 6]  OutputSizes=1
  Selector3 : Selector  InputPortWidth=12  IndexOptions=Index vector (dialog)  Indices=[12]  OutputSizes=1
  Selector4 : Selector  InputPortWidth=12  IndexOptions=Index vector (dialog)  Indices=[3]  OutputSizes=1
  tau_thrust : Outport
  tau_yaw : Outport  Port=2
  tau_pitch : Outport  Port=3
  tau_roll : Outport  Port=4
  wires:
  Attitude controller/2(tau_Pitch) -> Mux/3
  Selector3/1 -> Altitude Controller/1(z)
  Selector4/1 -> Altitude Controller/2(vz)
  Attitude controller/3(tau_Roll) -> Mux/4
  Attitude controller/1(tau_Yaw) -> Mux/2
  Altitude Controller/1(tau_Thrust) -> Mux/1
  Demux/2 -> tau_yaw/1  "-0.1 ~ 0.1"
  Mux/1 -> Demux/1
  Demux/1 -> tau_thrust/1  "0~1"
  Demux/3 -> tau_pitch/1  "-0.2 ~ 0.2"
  Demux/4 -> tau_roll/1  "-0.2 ~ 0.2"
  [x] -> Selector4/1, Selector3/1
  x/1 -> [x]
  des_roll/1 -> ?
  des_pitch/1 -> ?
  des_yawrate/1 -> ?
  des_alt/1 -> Altitude Controller/3(des_alt)
  Manual Switch/1 -> Add1/1
  Constant1/1 -> Manual Switch1/2
  Band-Limited White Noise1/1 -> Manual Switch1/1
  Band-Limited White Noise/1 -> Manual Switch/1
  Manual Switch1/1 -> Add/2
  Constant/1 -> Manual Switch/2
  Selector1/1 -> Add1/2
  [x] -> Selector2/1, Selector1/1
  Selector2/1 -> Add/1
  Add1/1 -> Delay/1
  Add/1 -> Delay1/1
  Delay/1 -> [RPY]
  Delay1/1 -> [pqr]
  [pqr] -> ?
  [RPY] -> ?
